simulink model "acmi7"  (Simulink 6.5)
settings: Solver=ode23t  StartTime=0.0  StopTime=2  RelTol=1e-3
undefined symbols (not defined in the file): powergui
libraries: powerlib x12
settings Model: Creator=RS  LastModifiedBy=RS

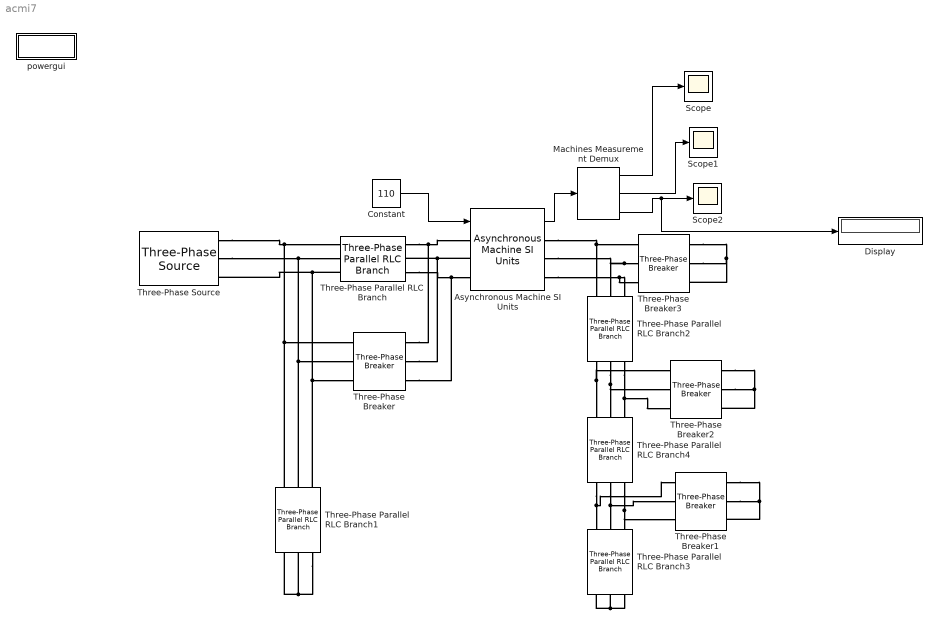
== system acmi7 ==
  Asynchronous Machine SI Units : powerlib/Machines/Asynchronous Machine SI Units  DialogController=PMDialogs.PMDefaultMaskDlg  SystemSampleTime=-1  PresetModel=No  MechanicalLoad=Torque Tm  ShowDetailedParameters=on  RotorType=Wound  ReferenceFrame=Stationary  NominalParameters="[6.5*746    380   50]"  Stator="[0.63   0.00496]"  Rotor="[1.094   0.00496]"  Lm=0.105  Mechanical=[0.05 0.005752 2]  PolePairs=2  InitialConditions="[ 1,0   0,0,0   0,0,0 ]"  Units=1  LoadFlowParameters=0  SimulateSaturation=off  Saturation=[9.9249,19.6672,38.0377,51.3988,69.2824,105.1337,152.5532,214.2421,303.1917;230, 322, 414, 460, 506, 552, 598, 644, 690]
  Constant : Constant  Value=110  OutDataType=sfix(16)  ConRadixGroup=Use specified scaling  OutScaling=2^0  SampleTime=inf  FramePeriod=inf
  Display : Display
  Machines Measurement Demux : powerlib/Machines/Machines Measurement Demux  DialogController=PMDialogs.PMDefaultMaskDlg  SystemSampleTime=-1  machType=Asynchronous  ssm1=on  ssm2=on  ssm3=on  ssm4=on  ssm5=on  ssm6=on  sm1=off  sm2=off  sm3=off  sm4=off  sm5=off  sm6=off  sm7=off  sm8=on  sm9=off  sm10=off  sm11=off  sm115=off  sm12=off  sm13=off  sm14=off  asm1=off  asm2=off  asm3=off  asm4=off  asm5=on  asm6=off  asm7=off  asm8=off  asm9=on  asm10=on  asm11=off  pmsm1=on  pmsm2=on  pmsm3=on  pmsm4=off  pmsm5=on  pmsm6=on  pmsm7=on  lastType=1
  Scope : Scope
      settings: MaxDataPoints=10000000  SampleInput=on  SampleTime=10e-6
  Scope1 : Scope
      settings: MaxDataPoints=10000000  SampleInput=on  SampleTime=10e-6
  Scope2 : Scope
      settings: TimeRange=1  YMin=10.8893  YMax=10.893  SaveName=ScopeData2  MaxDataPoints=10000000  SampleInput=on  SampleTime=10e-6
  Three-Phase Parallel RLC Branch : powerlib/Elements/Three-Phase Parallel RLC Branch  Orientation=left  DialogController=PMDialogs.PMDefaultMaskDlg  PhysicalDomain=powersysdomain  SubClassName=unknown  LeftPortType=p1  RightPortType=p1  LConnTagsString=A|B|C  RConnTagsString=A|B|C  BranchType=R  Resistance=8  Inductance=1e-3  Capacitance=400e-6  Measurements=None
  Three-Phase Parallel RLC Branch1 : powerlib/Elements/Three-Phase Parallel RLC Branch  Orientation=up  DialogController=PMDialogs.PMDefaultMaskDlg  PhysicalDomain=powersysdomain  SubClassName=unknown  LeftPortType=p1  RightPortType=p1  LConnTagsString=A|B|C  RConnTagsString=A|B|C  BranchType=R  Resistance=1000000  Inductance=1e-3  Capacitance=90e-6  Measurements=None
  Three-Phase Parallel RLC Branch2 : powerlib/Elements/Three-Phase Parallel RLC Branch  Orientation=up  DialogController=PMDialogs.PMDefaultMaskDlg  PhysicalDomain=powersysdomain  SubClassName=unknown  LeftPortType=p1  RightPortType=p1  LConnTagsString=A|B|C  RConnTagsString=A|B|C  BranchType=R  Resistance=1  Inductance=1e-3  Capacitance=400e-6  Measurements=None
  Three-Phase Parallel RLC Branch3 : powerlib/Elements/Three-Phase Parallel RLC Branch  Orientation=up  DialogController=PMDialogs.PMDefaultMaskDlg  PhysicalDomain=powersysdomain  SubClassName=unknown  LeftPortType=p1  RightPortType=p1  LConnTagsString=A|B|C  RConnTagsString=A|B|C  BranchType=R  Resistance=0.5006  Inductance=1e-3  Capacitance=400e-6  Measurements=None
  Three-Phase Parallel RLC Branch4 : powerlib/Elements/Three-Phase Parallel RLC Branch  Orientation=up  DialogController=PMDialogs.PMDefaultMaskDlg  PhysicalDomain=powersysdomain  SubClassName=unknown  LeftPortType=p1  RightPortType=p1  LConnTagsString=A|B|C  RConnTagsString=A|B|C  BranchType=R  Resistance=0.5  Inductance=1e-3  Capacitance=400e-6  Measurements=None
  Three-Phase Breaker : powerlib/Elements/Three-Phase Breaker  DialogController=PMDialogs.PMDefaultMaskDlg  SystemSampleTime=-1  InitialState=closed  SwitchA=on  SwitchB=on  SwitchC=on  SwitchTimes=5  External=off  BreakerResistance=0.001  SnubberResistance=1e6  SnubberCapacitance=inf  Measurements=None
  Three-Phase Breaker1 : powerlib/Elements/Three-Phase Breaker  DialogController=PMDialogs.PMDefaultMaskDlg  SystemSampleTime=-1  InitialState=open  SwitchA=on  SwitchB=on  SwitchC=on  SwitchTimes=3  External=off  BreakerResistance=0.001  SnubberResistance=1e6  SnubberCapacitance=inf  Measurements=None
  Three-Phase Breaker2 : powerlib/Elements/Three-Phase Breaker  DialogController=PMDialogs.PMDefaultMaskDlg  SystemSampleTime=-1  InitialState=open  SwitchA=on  SwitchB=on  SwitchC=on  SwitchTimes=3  External=off  BreakerResistance=0.001  SnubberResistance=1e6  SnubberCapacitance=inf  Measurements=None
  Three-Phase Breaker3 : powerlib/Elements/Three-Phase Breaker  DialogController=PMDialogs.PMDefaultMaskDlg  SystemSampleTime=-1  InitialState=open  SwitchA=on  SwitchB=on  SwitchC=on  SwitchTimes=1.5  External=off  BreakerResistance=0.001  SnubberResistance=1e6  SnubberCapacitance=inf  Measurements=None
  Three-Phase Source : powerlib/Electrical Sources/Three-Phase Source  DialogController=PMDialogs.PMDefaultMaskDlg  SystemSampleTime=-1  Voltage=380  PhaseAngle=0  Frequency=50  InternalConnection=Yg  SpecifyImpedance=off  Resistance=0.0001  Inductance=0.0001  ShortCircuitLevel=100e6  BaseVoltage=25e3  XRratio=7
  powergui : Subsystem  AncestorBlock=powerlib/powergui  InitFcn=powergui( 'InitFcn_Callback' , gcb , 0 , [ ] );  mask(PSB option menu block){SimulationMode=Continuous, SampleTime=50e-6, echomessages=off, RestoreLinks=warning, x0status=blocks, Frange=[0:2:500], Ylog=off, Xlog=on, ShowGrid=off, save=off, variable=ZData, structure=, ZoomFFT=on, StartTime=0.0, cycles=1, DisplayStyle=1, fundamental=60, FreqAxis=off, MaxFrequency=1000, frequencyindice=50, frequencyindicesteady=1, RmsSteady=1, display=off, Ts=0, frequency=60, methode=off, HookPort=off, Interpol=off}
      mask prompts: SimulationMode "Simulation mode"; SampleTime "Sample time Ts (when simulation mode is Discrete) (s)"; echomessages "Echo  Messages"; RestoreLinks "Restore disabled links"; x0status "Initial electrical states status"; Frange "Impedance tool: Frequency Range"; Ylog "Impedance tool: Log impedance"; Xlog "Impedance tool: log Frequency"; ShowGrid "Impedance tool: grid"; save "Impedance tool: Save Data To Workspace"; variable "Impedance tool: Variable Name"; structure "Structure Name (PSBFFTSCOPE)"; ZoomFFT "ZoomFFT (PSBFFTSCOPE)"; StartTime "Start Time (PSBFFTSCOPE)"; cycles "Cycles (PSBFFTSCOPE)"; DisplayStyle "Display style (PSBFFTSCOPE)"; fundamental "Fundamental (PSBFFTSCOPE)"; FreqAxis "Frequency Axis (PSBFFTSCOPE)"; MaxFrequency "Max Frequency (PSBFFTSCOPE)"; frequencyindice "Load flow frequency (Hz)"; frequencyindicesteady "Frequency indice (STEADYSTATE)"; RmsSteady "RMS display (STEADYSTATE)"; display "Display Results"; Ts "OBSOLETE 1"; frequency "Phasor frequency (Hz)"; methode "Phasor simulation"; HookPort "Hook port"; Interpol "Interpolate"
      mask init:
      | powerlibroot = which('powersysdomain');
      | PSBroot = powerlibroot(1:end-16);
      | %
      | switch SimulationMode
      | 	case 1
      | 		message=sprintf('Continuous');
      | 	case 2
      |         SampleTimeeval=evalin('base',SampleTime,'NaN');
      |         if isnan(SampleTimeeval)
      |             message=sprintf('Warning !!,\nUndefined sample time');
      |         else
      |             message=sprintf('Discrete,\nTs = %.4g s.',SampleTimeeval);
      |         end
      | 	case 3
      | 		message=sprintf('Phasors');
      | end
      | if strcmp(bdroot,'powerlib')
      |   message='powergui';
      | end
      | power_initmask();
      settings: CopyFcn=powergui( 'Copy_Callback' , gcb , 0 , [ ] );  ModelCloseFcn=powergui( 'CloseButton_Callback' , gcb , [ ] , [ ] );  PreSaveFcn=powergui( 'CloseButton_Callback' , gcb , [ ] , [ ] );  NameChangeFcn=powergui( 'NameChangeFcn_Callback' , gcb , 0 , [ ] );
      settings: DeleteFcn=|
      | powergui( 'Copy_Callback' , gcb , 1 , [ ] );
      | powergui( 'CloseButton_Callback' , gcb , [ ] , [ ] );
      settings: OpenFcn=|
      | if (power_openblockproxy ('secondary'))
      | powergui(gcb,'PM')
      | end;
      mask Help: web(psbhelp)
      mask StyleString: popup(Continuous|Discrete|Phasor),edit,checkbox,popup(yes|warning|no),popup(blocks|steady|zero),edit,checkbox,checkbox,checkbox,checkbox,edit,edit,checkbox,edit,edit,edit,edit,checkbox,edit,edit,edit,edit,checkbox,edit,edit,checkbox,checkbox,checkbox
      mask CallbackString: ||||||||||||||||||||||||||powergui('HookPort',[],[],gcb);|
      mask Display: disp(message)
  wires:
  Constant/1 -> Asynchronous Machine SI Units/1
  Asynchronous Machine SI Units/1 -> Machines Measurement Demux/1
  Machines Measurement Demux/3 -> Scope2/1, Display/1
  Machines Measurement Demux/2 -> Scope1/1
  Machines Measurement Demux/1 -> Scope/1
  connections:
  Three-Phase Parallel RLC Branch1/RConn1 -- Three-Phase Source/RConn1 -- Three-Phase Parallel RLC Branch/RConn1 -- Three-Phase Breaker/LConn1
  Three-Phase Parallel RLC Branch1/RConn2 -- Three-Phase Source/RConn2 -- Three-Phase Parallel RLC Branch/RConn2 -- Three-Phase Breaker/LConn2
  Three-Phase Parallel RLC Branch1/RConn3 -- Three-Phase Parallel RLC Branch/RConn3 -- Three-Phase Source/RConn3 -- Three-Phase Breaker/LConn3
  Three-Phase Parallel RLC Branch/LConn1 -- Asynchronous Machine SI Units/LConn1 -- Three-Phase Breaker/RConn1
  Asynchronous Machine SI Units/LConn2 -- Three-Phase Parallel RLC Branch/LConn2 -- Three-Phase Breaker/RConn2
  Three-Phase Parallel RLC Branch/LConn3 -- Asynchronous Machine SI Units/LConn3 -- Three-Phase Breaker/RConn3
  Three-Phase Parallel RLC Branch1/LConn3 -- Three-Phase Parallel RLC Branch1/LConn1 -- Three-Phase Parallel RLC Branch1/LConn2
  Asynchronous Machine SI Units/RConn1 -- Three-Phase Parallel RLC Branch2/RConn1 -- Three-Phase Breaker3/LConn1
  Three-Phase Breaker3/LConn2 -- Asynchronous Machine SI Units/RConn2 -- Three-Phase Parallel RLC Branch2/RConn2
  Asynchronous Machine SI Units/RConn3 -- Three-Phase Parallel RLC Branch2/RConn3 -- Three-Phase Breaker3/LConn3
  Three-Phase Parallel RLC Branch2/LConn1 -- Three-Phase Parallel RLC Branch4/RConn1 -- Three-Phase Breaker2/LConn1
  Three-Phase Parallel RLC Branch2/LConn2 -- Three-Phase Parallel RLC Branch4/RConn2 -- Three-Phase Breaker2/LConn2
  Three-Phase Parallel RLC Branch2/LConn3 -- Three-Phase Parallel RLC Branch4/RConn3 -- Three-Phase Breaker2/LConn3
  Three-Phase Parallel RLC Branch4/LConn1 -- Three-Phase Parallel RLC Branch3/RConn1 -- Three-Phase Breaker1/LConn1
  Three-Phase Parallel RLC Branch4/LConn2 -- Three-Phase Parallel RLC Branch3/RConn2 -- Three-Phase Breaker1/LConn2
  Three-Phase Parallel RLC Branch4/LConn3 -- Three-Phase Parallel RLC Branch3/RConn3 -- Three-Phase Breaker1/LConn3
  Three-Phase Parallel RLC Branch3/LConn3 -- Three-Phase Parallel RLC Branch3/LConn1 -- Three-Phase Parallel RLC Branch3/LConn2
  Three-Phase Breaker3/RConn1 -- Three-Phase Breaker3/RConn3 -- Three-Phase Breaker3/RConn2
  Three-Phase Breaker2/RConn1 -- Three-Phase Breaker2/RConn3 -- Three-Phase Breaker2/RConn2
  Three-Phase Breaker1/RConn1 -- Three-Phase Breaker1/RConn3 -- Three-Phase Breaker1/RConn2

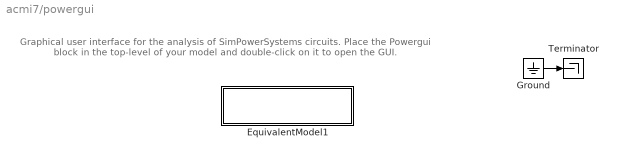
== system acmi7/powergui ==
  note: Graphical user interface for the analysis of  SimPowerSystems circuits.
      | Place the Powergui block in the top-level of your model and double-click
      | on it to open the GUI.
  EquivalentModel1 : Subsystem
      mask init:
      | SPS = get_param(gcbh,'UserData');
      | if isempty(SPS)
      |     A=0;
      |     B=0;
      |     C=0;
      |     D=0;
      |     x0=0;
      |     SwitchResistance=1;
      |     SwitchType=1;
      |     SwitchGateInitialValue=1;
      |     OutputsToResetToZero=1;
      | else
      | 	A=SPS.A;
      |     B=SPS.B;
      |     C=SPS.C;
      |     D=SPS.D;
      |     x0=SPS.x0;
      |     SwitchResistance=SPS.SwitchResistance;
      |     SwitchType=SPS.SwitchType;
      |     SwitchGateInitialValue=SPS.SwitchGateInitialValue;
      |     OutputsToResetToZero=SPS.YSwitchCurrent;
      | end
      mask Display:
      | color('blue')
      | disp('EQUIVALENT CIRCUIT')
  Ground : Ground
  Terminator : Terminator
  wires:
  Ground/1 -> Terminator/1

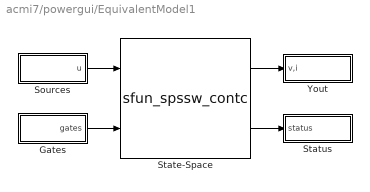
== system acmi7/powergui/EquivalentModel1 ==
  Gates : Subsystem
  Sources : Subsystem
  State-Space : S-Function  FunctionName=sfun_spssw_contc  Parameters=A, B, C, D, x0, SwitchResistance ,SwitchType, SwitchGateInitialValue, OutputsToResetToZero
  Status : Subsystem
  Yout : Subsystem
  wires:
  Gates/1(gates) -> State-Space/2
  Sources/1(u) -> State-Space/1
  State-Space/2 -> Status/1(status)
  State-Space/1 -> Yout/1(v,i)

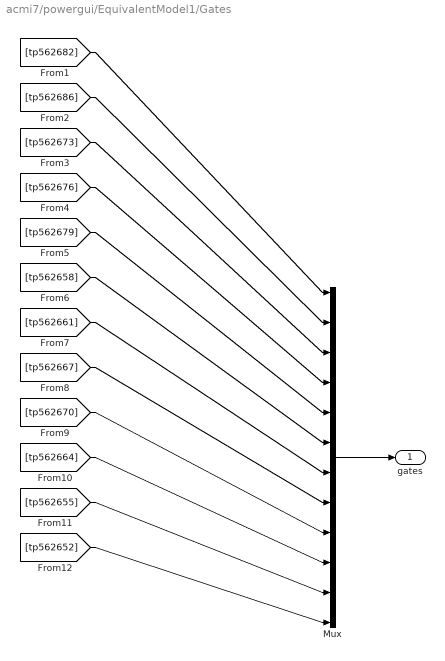
== system acmi7/powergui/EquivalentModel1/Gates ==
  Mux : Mux  Inputs=[1 1 1 1 1 1 1 1 1 1 1 1]
  gates : Outport
  wires:
  Mux/1 -> gates/1
  [tp562682] -> Mux/1
  [tp562686] -> Mux/2
  [tp562673] -> Mux/3
  [tp562676] -> Mux/4
  [tp562679] -> Mux/5
  [tp562658] -> Mux/6
  [tp562661] -> Mux/7
  [tp562667] -> Mux/8
  [tp562670] -> Mux/9
  [tp562664] -> Mux/10
  [tp562655] -> Mux/11
  [tp562652] -> Mux/12

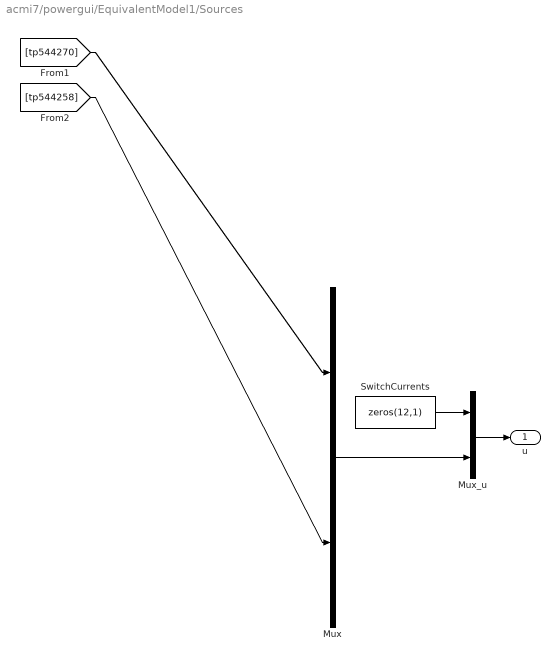
== system acmi7/powergui/EquivalentModel1/Sources ==
  Mux : Mux  Inputs=[4 3]
  Mux_u : Mux  Inputs=[12 7]
  SwitchCurrents : Constant  Value=zeros(12,1)  OutDataType=sfix(16)  ConRadixGroup=Use specified scaling  OutScaling=2^0  SampleTime=inf  FramePeriod=inf
  u : Outport
  wires:
  Mux/1 -> Mux_u/2
  SwitchCurrents/1 -> Mux_u/1
  Mux_u/1 -> u/1
  [tp544270] -> Mux/1
  [tp544258] -> Mux/2

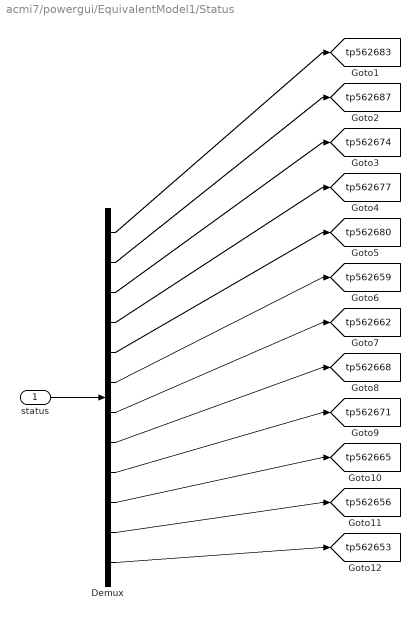
== system acmi7/powergui/EquivalentModel1/Status ==
  status : Inport
  Demux : Demux  Outputs=[1 1 1 1 1 1 1 1 1 1 1 1]
  tag scope: tp562653=global, tp562656=global, tp562659=global, tp562662=global, tp562665=global, tp562668=global, tp562671=global, tp562674=global, tp562677=global, tp562680=global, tp562683=global, tp562687=global
  wires:
  status/1 -> Demux/1
  Demux/1 -> [tp562683]
  Demux/2 -> [tp562687]
  Demux/3 -> [tp562674]
  Demux/4 -> [tp562677]
  Demux/5 -> [tp562680]
  Demux/6 -> [tp562659]
  Demux/7 -> [tp562662]
  Demux/8 -> [tp562668]
  Demux/9 -> [tp562671]
  Demux/10 -> [tp562665]
  Demux/11 -> [tp562656]
  Demux/12 -> [tp562653]

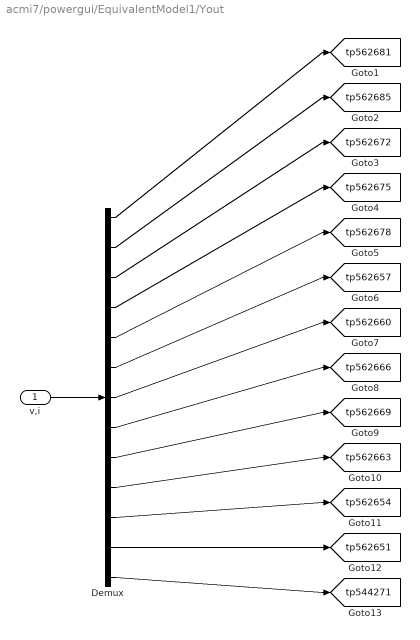
== system acmi7/powergui/EquivalentModel1/Yout ==
  v,i : Inport
  Demux : Demux  Outputs=[1 1 1 1 1 1 1 1 1 1 1 1 4]
  tag scope: tp544271=global, tp562651=global, tp562654=global, tp562657=global, tp562660=global, tp562663=global, tp562666=global, tp562669=global, tp562672=global, tp562675=global, tp562678=global, tp562681=global, tp562685=global
  wires:
  v,i/1 -> Demux/1
  Demux/1 -> [tp562681]
  Demux/2 -> [tp562685]
  Demux/3 -> [tp562672]
  Demux/4 -> [tp562675]
  Demux/5 -> [tp562678]
  Demux/6 -> [tp562657]
  Demux/7 -> [tp562660]
  Demux/8 -> [tp562666]
  Demux/9 -> [tp562669]
  Demux/10 -> [tp562663]
  Demux/11 -> [tp562654]
  Demux/12 -> [tp562651]
  Demux/13 -> [tp544271]
